simulink model "Quadcopter_V5"  (R2024a)
settings: Solver=ode4  StartTime=0.0  StopTime=inf  FixedStep=0.01  RelTol=1e-3
undefined symbols (not defined in the file): F, MIL, Severe
libraries: slpidlib x8, simulink_extras x4, aerolibpropulsion2 x4, aerolibwind2 x2, shared6dof x1, aerolibatmos2 x1, aerolibanimutils x1, sharedtransform x1, uavutilslib x1
(part 1 of 2)
settings Model: Creator=aceco  LastModifiedBy=Anthony

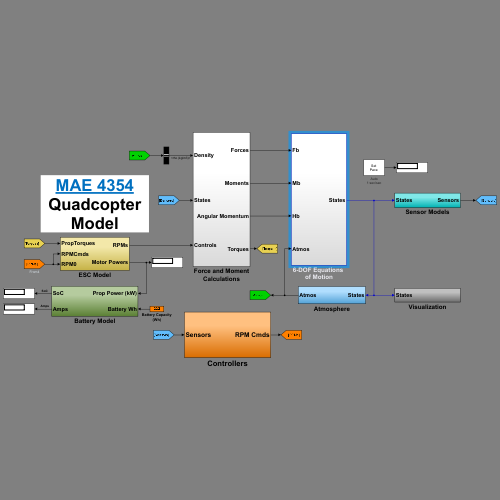
[thumbnail: Simulink's stored preview of the top-level diagram]
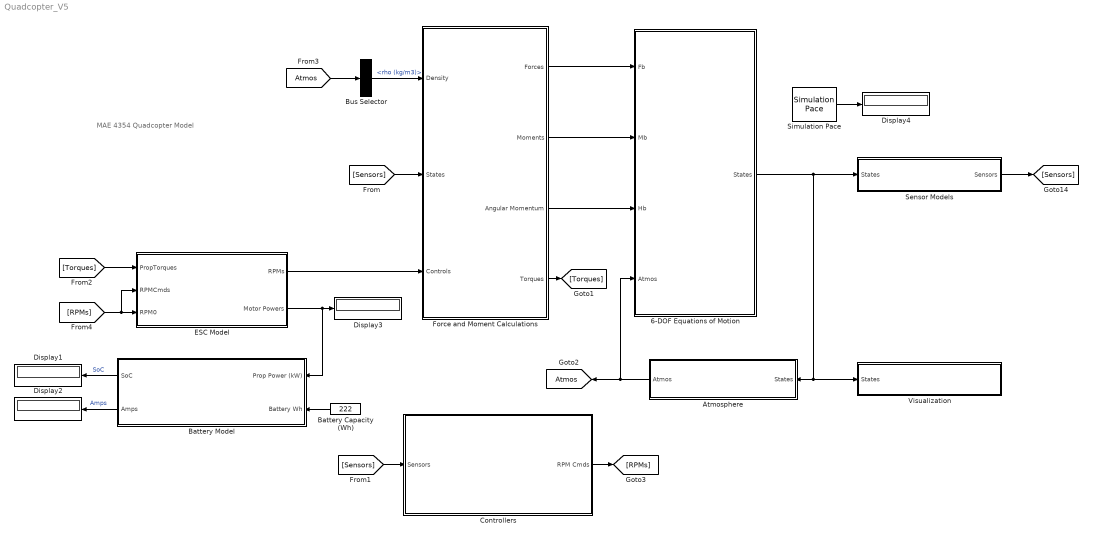
== system Quadcopter_V5 ==
  note: MAE 4354
      | Quadcopter Model
  6-DOF Equations of Motion : Subsystem
  Atmosphere : Subsystem
  Battery Capacity (Wh) : Constant  Value=222
  Battery Model : Subsystem
  Bus Selector : BusSelector  OutputSignals=rho (kg/m3)
  Controllers : Subsystem
  Display{1..4} (4 alike) : Display
  ESC Model : Subsystem
  Force and Moment Calculations : Subsystem
  Sensor Models : Subsystem
  Simulation Pace : aerolibanimutils/Simulation Pace  SimulationPace=1  SleepMode=Auto  OutputPaceError=on  SampleTime=-1
  Visualization : Subsystem
  tag scope: Atmos=global
  wires:
  Simulation Pace/1 -> Display4/1
  6-DOF Equations of Motion/1(States) -> Visualization/1(States), Atmosphere/1(States), Sensor Models/1(States)
  Force and Moment Calculations/1(Forces) -> 6-DOF Equations of Motion/1(Fb)
  Force and Moment Calculations/2(Moments) -> 6-DOF Equations of Motion/2(Mb)
  [Sensors] -> Force and Moment Calculations/2(States)
  ESC Model/1(RPMs) -> Force and Moment Calculations/3(Controls)
  [RPMs] -> ESC Model/2(RPMCmds), ESC Model/3(RPM0)
  Battery Model/2(Amps) -> Display2/1  "Amps"
  Battery Model/1(SoC) -> Display1/1  "SoC"
  Battery Capacity (Wh)/1 -> Battery Model/2(Battery Wh)
  ESC Model/2(Motor Powers) -> Display3/1, Battery Model/1(Prop Power (kW))
  Sensor Models/1(Sensors) -> [Sensors]
  [Sensors] -> Controllers/1(Sensors)
  Force and Moment Calculations/4(Torques) -> [Torques]
  [Torques] -> ESC Model/1(PropTorques)
  Atmosphere/1(Atmos) -> [Atmos], 6-DOF Equations of Motion/4(Atmos)
  Bus Selector/1 -> Force and Moment Calculations/1(Density)  "<rho (kg/m3)>"
  [Atmos] -> Bus Selector/1
  Force and Moment Calculations/3(Angular Momentum) -> 6-DOF Equations of Motion/3(Hb)
  Controllers/1(RPM Cmds) -> [RPMs]

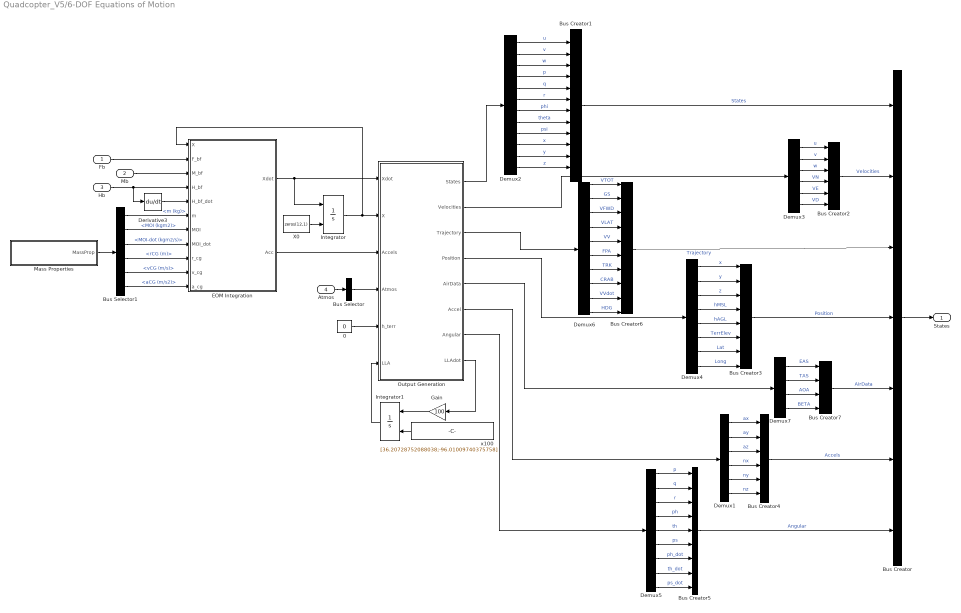
== system Quadcopter_V5/6-DOF Equations of Motion ==
  Fb : Inport
  Mb : Inport  Port=2
  Hb : Inport  Port=3
  Atmos : Inport  Port=4
  0 : Constant  Value=0
  Bus Creator : BusCreator  Inputs=7
  Bus Creator1 : BusCreator  Inputs=12
  Bus Creator2 : BusCreator  Inputs=6
  Bus Creator3 : BusCreator  Inputs=8
  Bus Creator4 : BusCreator  Inputs=6
  Bus Creator5 : BusCreator  Inputs=9
  Bus Creator6 : BusCreator  Inputs=10
  Bus Creator7 : BusCreator  Inputs=4
  Bus Selector : BusSelector  OutputSignals=V_wind (m/s),Om_wind (m/s),rho (kg/m3)  OutputAsBus=on
  Bus Selector1 : BusSelector  OutputSignals=m (kg),MOI (kgm2),MOI-dot (kgm2/s),rCG (m),vCG (m/s),aCG (m/s2)
  Demux1 : Demux  Outputs=6
  Demux2 : Demux  Outputs=12
  Demux3 : Demux  Outputs=6
  Demux4 : Demux  Outputs=8
  Demux5 : Demux  Outputs=9
  Demux6 : Demux  Outputs=10
  Demux7 : Demux
  Derivative3 : Derivative
  EOM Integration : MATLAB Function  TreatAsAtomicUnit=on
  Gain : Gain  Gain=100
  Integrator : Integrator  InitialConditionSource=external
  Integrator1 : Integrator  InitialConditionSource=external
  Mass Properties : Subsystem
  Output Generation : MATLAB Function  TreatAsAtomicUnit=on
  X0 : Constant  Value=zeros(12,1)
  x100 : Constant  Value=[36.20728752088038;-96.01009740375758]
  States : Outport  VectorParamsAs1DForOutWhenUnconnected=off
  wires:
  Bus Creator/1 -> States/1
  X0/1 -> Integrator/2
  Fb/1 -> EOM Integration/2(F_bf)
  Integrator/1 -> EOM Integration/1(X), Output Generation/2(X)
  Mb/1 -> EOM Integration/3(M_bf)
  Demux2/1 -> Bus Creator1/1  "u"
  Demux2/2 -> Bus Creator1/2  "v"
  Demux2/3 -> Bus Creator1/3  "w"
  Bus Creator1/1 -> Bus Creator/1  "States"
  Bus Creator2/1 -> Bus Creator/2  "Velocities"
  Demux3/3 -> Bus Creator2/3  "w"
  Demux3/2 -> Bus Creator2/2  "v"
  Demux3/1 -> Bus Creator2/1  "u"
  Demux2/4 -> Bus Creator1/4  "p"
  Demux2/5 -> Bus Creator1/5  "q"
  Demux2/6 -> Bus Creator1/6  "r"
  Demux3/4 -> Bus Creator2/4  "VN"
  Demux3/5 -> Bus Creator2/5  "VE"
  Demux3/6 -> Bus Creator2/6  "VD"
  Demux4/1 -> Bus Creator3/1  "x"
  Demux4/2 -> Bus Creator3/2  "y"
  Demux4/3 -> Bus Creator3/3  "z"
  Bus Creator3/1 -> Bus Creator/4  "Position"
  Demux1/1 -> Bus Creator4/1  "ax"
  Demux1/2 -> Bus Creator4/2  "ay"
  Demux1/3 -> Bus Creator4/3  "az"
  Demux1/4 -> Bus Creator4/4  "nx"
  Demux1/5 -> Bus Creator4/5  "ny"
  Demux1/6 -> Bus Creator4/6  "nz"
  Bus Creator4/1 -> Bus Creator/6  "Accels"
  Demux5/1 -> Bus Creator5/1  "p"
  Demux5/2 -> Bus Creator5/2  "q"
  Demux5/3 -> Bus Creator5/3  "r"
  Demux5/4 -> Bus Creator5/4  "ph"
  Demux5/5 -> Bus Creator5/5  "th"
  Demux5/6 -> Bus Creator5/6  "ps"
  Demux5/7 -> Bus Creator5/7  "ph_dot"
  Demux5/8 -> Bus Creator5/8  "th_dot"
  Demux5/9 -> Bus Creator5/9  "ps_dot"
  Bus Creator5/1 -> Bus Creator/7  "Angular"
  Bus Creator7/1 -> Bus Creator/5  "AirData"
  Bus Creator6/1 -> Bus Creator/3  "Trajectory"
  EOM Integration/1(Xdot) -> Integrator/1, Output Generation/1(Xdot)
  Demux4/8 -> Bus Creator3/8  "Long"
  Demux4/7 -> Bus Creator3/7  "Lat"
  Demux4/6 -> Bus Creator3/6  "TerrElev"
  Demux4/5 -> Bus Creator3/5  "hAGL"
  Demux4/4 -> Bus Creator3/4  "hMSL"
  EOM Integration/2(Acc) -> Output Generation/3(Accels)
  Atmos/1 -> Bus Selector/1
  Bus Selector/1 -> Output Generation/4(Atmos)
  Output Generation/8(LLAdot) -> Gain/1
  Integrator1/1 -> Output Generation/6(LLA)
  x100/1 -> Integrator1/2
  Output Generation/1(States) -> Demux2/1
  Demux2/7 -> Bus Creator1/7  "phi"
  Demux2/8 -> Bus Creator1/8  "theta"
  Demux2/9 -> Bus Creator1/9  "psi"
  Demux2/10 -> Bus Creator1/10  "x"
  Demux2/11 -> Bus Creator1/11  "y"
  Demux2/12 -> Bus Creator1/12  "z"
  Output Generation/2(Velocities) -> Demux3/1
  Demux6/7 -> Bus Creator6/7  "TRK"
  Demux6/8 -> Bus Creator6/8  "CRAB"
  Demux6/9 -> Bus Creator6/9  "VVdot"
  Demux6/1 -> Bus Creator6/1  "VTOT"
  Demux6/4 -> Bus Creator6/4  "VLAT"
  Demux6/5 -> Bus Creator6/5  "VV"
  Demux6/3 -> Bus Creator6/3  "VFWD"
  Demux6/2 -> Bus Creator6/2  "GS"
  Demux6/6 -> Bus Creator6/6  "FPA"
  Demux6/10 -> Bus Creator6/10  "HDG"
  Output Generation/3(Trajectory) -> Demux6/1
  Output Generation/4(Position) -> Demux4/1
  Demux7/4 -> Bus Creator7/4  "BETA"
  Demux7/1 -> Bus Creator7/1  "EAS"
  Demux7/2 -> Bus Creator7/2  "TAS"
  Demux7/3 -> Bus Creator7/3  "AOA"
  Output Generation/5(AirData) -> Demux7/1
  Output Generation/6(Accel) -> Demux1/1
  Output Generation/7(Angular) -> Demux5/1
  0/1 -> Output Generation/5(h_terr)
  Gain/1 -> Integrator1/1
  Hb/1 -> EOM Integration/4(H_bf), Derivative3/1
  Derivative3/1 -> EOM Integration/5(H_bf_dot)
  Mass Properties/1(MassProp) -> Bus Selector1/1
  Bus Selector1/1 -> EOM Integration/6(m)  "<m (kg)>"
  Bus Selector1/4 -> EOM Integration/9(r_cg)  "<rCG (m)>"
  Bus Selector1/5 -> EOM Integration/10(v_cg)  "<vCG (m/s)>"
  Bus Selector1/6 -> EOM Integration/11(a_cg)  "<aCG (m/s2)>"
  Bus Selector1/2 -> EOM Integration/7(MOI)  "<MOI (kgm2)>"
  Bus Selector1/3 -> EOM Integration/8(MOI_dot)  "<MOI-dot (kgm2/s)>"

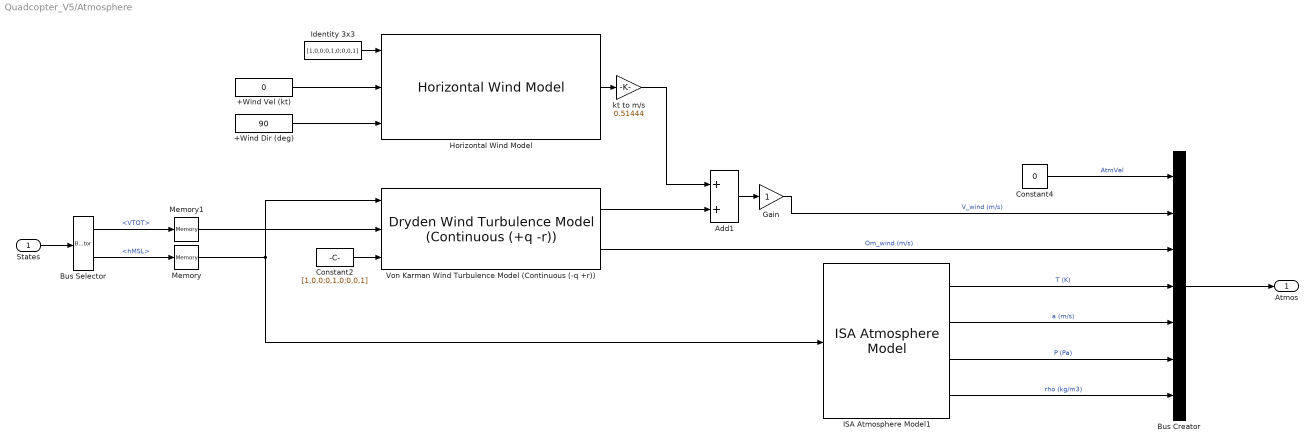
== system Quadcopter_V5/Atmosphere ==
  States : Inport
  +Wind Dir (deg) : Constant  Value=90
  +Wind Vel (kt) : Constant  Value=0
  Add1 : Sum  Inputs=2
  Bus Creator : BusCreator  Inputs=7
  Bus Selector : BusSelector  OutputSignals=Trajectory.VTOT,Position.hMSL
  Constant2 : Constant  Value=[1,0,0;0,1,0;0,0,1]
  Constant4 : Constant  Value=0
  Gain : Gain
  Horizontal Wind Model : aerolibwind2/Horizontal Wind Model  units=English (Velocity in kts)  Vw_source=External  Vwind=Init.WindSpd  W_source=External  Wdeg=Init.WindDir
  ISA Atmosphere Model1 : aerolibatmos2/ISA Atmosphere Model  useExtended=off  action=Warning  custom=off  viscosityOut=off  g=9.80665  gamma=1.4  R=287.0531  L=0.0065  h_trop=11000  h_strat=20000  rho0=1.225  P0=101325  T0=288.15  h0=0  S=110.4  Tref=273.15  muref=1.716e-5
  Identity 3x3 : Constant  Value=[1,0,0;0,1,0;0,0,1]
  Memory : Memory
  Memory1 : Memory
  Von Karman Wind Turbulence Model (Continuous (-q +r)) : aerolibwind2/Dryden Wind Turbulence Model  (Continuous (+q -r))  units=Metric (MKS)  spec=MIL-F-8785C  model=Continuous Von Karman (-q +r)  W20=3  Wdeg=90  TurbProb=10^-5 - Severe  L_high=762  Wingspan=2  ts=0.2  Seed=[23341 23342 23343 23344]  T_on=off
  kt to m/s : Gain  Gain=0.51444
  Atmos : Outport  VectorParamsAs1DForOutWhenUnconnected=off
  wires:
  States/1 -> Bus Selector/1
  Bus Selector/2 -> Memory/1  "<hMSL>"
  Horizontal Wind Model/1 -> kt to m/s/1
  Add1/1 -> Gain/1
  ISA Atmosphere Model1/1 -> Bus Creator/4  "T (K)"
  ISA Atmosphere Model1/2 -> Bus Creator/5  "a (m/s)"
  ISA Atmosphere Model1/3 -> Bus Creator/6  "P (Pa)"
  ISA Atmosphere Model1/4 -> Bus Creator/7  "rho (kg/m3)"
  Bus Creator/1 -> Atmos/1
  Von Karman Wind Turbulence Model (Continuous (-q +r))/1 -> Add1/2
  Von Karman Wind Turbulence Model (Continuous (-q +r))/2 -> Bus Creator/3  "Om_wind (m/s)"
  Constant4/1 -> Bus Creator/1  "AtmVel"
  Identity 3x3/1 -> Horizontal Wind Model/1
  Constant2/1 -> Von Karman Wind Turbulence Model (Continuous (-q +r))/3
  kt to m/s/1 -> Add1/1
  +Wind Vel (kt)/1 -> Horizontal Wind Model/2
  +Wind Dir (deg)/1 -> Horizontal Wind Model/3
  Bus Selector/1 -> Memory1/1  "<VTOT>"
  Gain/1 -> Bus Creator/2  "V_wind (m/s)"
  Memory/1 -> Von Karman Wind Turbulence Model (Continuous (-q +r))/1, ISA Atmosphere Model1/1
  Memory1/1 -> Von Karman Wind Turbulence Model (Continuous (-q +r))/2

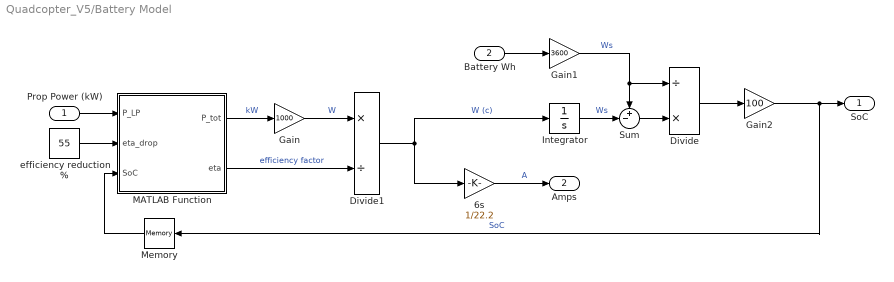
== system Quadcopter_V5/Battery Model ==
  Prop Power (kW) : Inport
  Battery Wh : Inport  Port=2
  6s : Gain  Gain=1/22.2
  Divide : Product  Inputs=/*
  Divide1 : Product  Inputs=*/
  Gain : Gain  Gain=1000
  Gain1 : Gain  Gain=3600
  Gain2 : Gain  Gain=100
  Integrator : Integrator
  MATLAB Function : MATLAB Function  TreatAsAtomicUnit=on
  Memory : Memory  InitialCondition=100
  Sum : Sum  Inputs=+-|
  efficiency reduction % : Constant  Value=55
  SoC : Outport
  Amps : Outport  Port=2
  wires:
  Battery Wh/1 -> Gain1/1
  6s/1 -> Amps/1  "A"
  Prop Power (kW)/1 -> MATLAB Function/1(P_LP)
  MATLAB Function/1(P_tot) -> Gain/1  "kW"
  Sum/1 -> Divide/2
  Integrator/1 -> Sum/2  "Ws"
  Divide/1 -> Gain2/1
  Gain2/1 -> Memory/1, SoC/1  "SoC"
  Divide1/1 -> 6s/1, Integrator/1  "W (c)"
  Gain1/1 -> Sum/1, Divide/1  "Ws"
  Gain/1 -> Divide1/1  "W"
  MATLAB Function/2(eta) -> Divide1/2  "efficiency factor"
  Memory/1 -> MATLAB Function/3(SoC)
  efficiency reduction %/1 -> MATLAB Function/2(eta_drop)

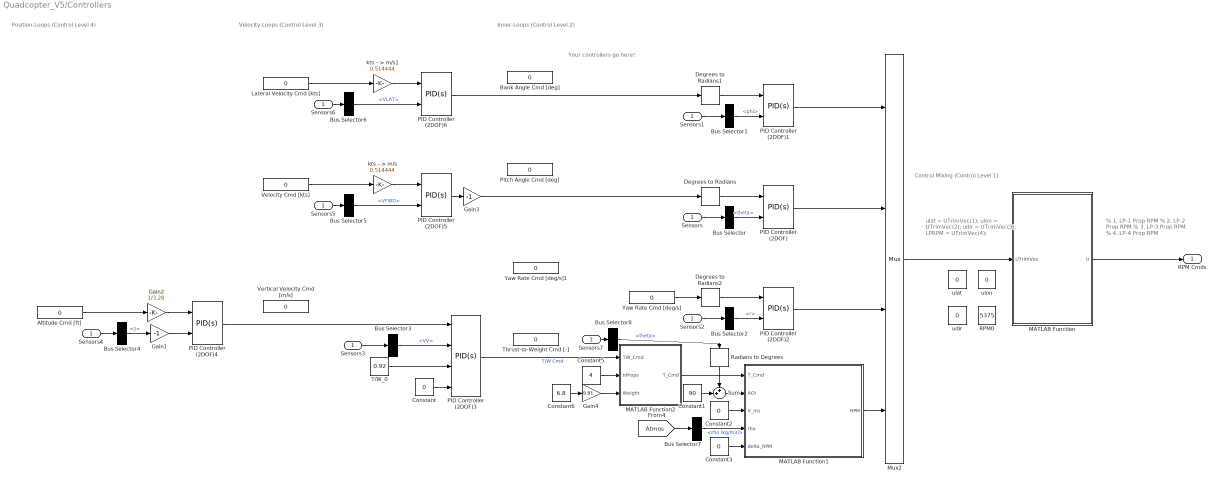
== system Quadcopter_V5/Controllers ==
  note: Inner-Loops (Control Level 2)
  note: Control Mixing (Control Level 1)
  note: Your controllers go here!
  note: ulat = UTrimVec(1);
      | ulon = UTrimVec(2);
      | udir = UTrimVec(3);
      | LPRPM = UTrimVec(4);
  note: % 1. LP-1 Prop RPM
      | % 2. LP-2 Prop RPM
      | % 3. LP-3 Prop RPM
      | % 4. LP-4 Prop RPM
  note: Velocity-Loops (Control Level 3)
  note: Position-Loops (Control Level 4)
  Sensors : Inport
  Altitude Cmd [ft] : Constant  Value=0
  Bank Angle Cmd [deg] : Constant  Value=0
  Bus Selector : BusSelector  OutputSignals=theta
  Bus Selector1 : BusSelector  OutputSignals=phi
  Bus Selector2 : BusSelector  OutputSignals=r
  Bus Selector3 : BusSelector  OutputSignals=VV
  Bus Selector4 : BusSelector  OutputSignals=z
  Bus Selector5 : BusSelector  OutputSignals=VFWD
  Bus Selector6 : BusSelector  OutputSignals=VLAT
  Bus Selector7 : BusSelector  OutputSignals=rho (kg/m3)
  Bus Selector8 : BusSelector  OutputSignals=theta
  Constant : Constant  Value=0
  Constant1 : Constant  Value=90
  Constant2 : Constant  Value=0
  Constant3 : Constant  Value=0
  Constant5 : Constant  Value=4
  Constant6 : Constant  Value=6.8
  Degrees to Radians : simulink_extras/Transformations/Degrees to Radians
  Degrees to Radians1 : simulink_extras/Transformations/Degrees to Radians
  Degrees to Radians2 : simulink_extras/Transformations/Degrees to Radians
  Gain1 : Gain  Gain=-1
  Gain2 : Gain  Gain=1/3.28
  Gain3 : Gain  Gain=-1
  Gain4 : Gain  Gain=9.81
  Lateral Velocity Cmd [kts] : Constant  Value=0
  MATLAB Function : MATLAB Function  TreatAsAtomicUnit=on
  MATLAB Function1 : MATLAB Function  TreatAsAtomicUnit=on
  MATLAB Function2 : MATLAB Function  TreatAsAtomicUnit=on
  Mux2 : Mux
  PID Controller (2DOF) : slpidlib/PID Controller (2DOF)  Controller=PID  Form=Parallel  TimeDomain=Continuous-time  UseExternalTs=off  SampleTime=-1  IntegratorMethod=Forward Euler  FilterMethod=Forward Euler  ControllerParametersSource=internal  P=2  I=0.5  UseKiTs=off  D=1  UseExternalDerivativeSource=off  N=100  UseFilter=on  b=1  c=1  TunerSelectOption=Transfer Function Based (PID Tuner App)  InitialConditionSource=internal  InitialConditionForIntegrator=0  InitialConditionForFilter=0  DifferentiatorICPrevScaledInput=0  ExternalReset=none  TrackingMode=off  Kt=1  LimitOutput=on  SatLimitsSource=internal  UpperSaturationLimit=1  LowerSaturationLimit=-1  LinearizeAsGain=on  AntiWindupMode=clamping  Kb=1  LimitIntegrator=off  UpperIntegratorSaturationLimit=inf  LowerIntegratorSaturationLimit=-inf  POutMin=[]  POutMax=[]  IOutMin=[]  IOutMax=[]  DOutMin=[]  DOutMax=[]  NOutMin=[]  NOutMax=[]  bOutMin=[]  bOutMax=[]  cOutMin=[]  cOutMax=[]  SumOutMin=[]  SumOutMax=[]  SaturationOutMin=[]  SaturationOutMax=[]  PParamMin=[]  PParamMax=[]  IParamMin=[]  IParamMax=[]  DParamMin=[]  DParamMax=[]  NParamMin=[]  NParamMax=[]  bParamMin=[]  bParamMax=[]  cParamMin=[]  cParamMax=[]  KbParamMin=[]  KbParamMax=[]  KtParamMin=[]  KtParamMax=[]  KbOutMin=[]  KbOutMax=[]  KtOutMin=[]  KtOutMax=[]  IntegratorOutMin=[]  IntegratorOutMax=[]  FilterOutMin=[]  FilterOutMax=[]  SumI1OutMin=[]  SumI1OutMax=[]  SumI2OutMin=[]  SumI2OutMax=[]  SumI3OutMin=[]  SumI3OutMax=[]  SumI4OutMin=[]  SumI4OutMax=[]  SumDOutMin=[]  SumDOutMax=[]  Sum1OutMin=[]  Sum1OutMax=[]  Sum2OutMin=[]  Sum2OutMax=[]  Sum3OutMin=[]  Sum3OutMax=[]  DifferentiatorOutMin=[]  DifferentiatorOutMax=[]  FilterDiffOutCoefMin=[]  FilterDiffOutCoefMax=[]  ReciprocalOutMin=[]  ReciprocalOutMax=[]  SumDenOutMin=[]  SumDenOutMax=[]  SumNumOutMin=[]  SumNumOutMax=[]  DivideOutMin=[]  DivideOutMax=[]  UdiffTsProdOutMin=[]  UdiffTsProdOutMax=[]  NTsProdOutMin=[]  NTsProdOutMax=[]  UintegralTsProdOutMin=[]  UintegralTsProdOutMax=[]  UngainTsProdOutMin=[]  UngainTsProdOutMax=[]  ClampingZeroOutDataTypeStr=Inherit: Inherit via back propagation  ClampingZeroOutMin=[]  ClampingZeroOutMax=[]  FilterDenConstantOutDataTypeStr=Inherit: Inherit via back propagation  FilterDenConstantOutMin=[]  FilterDenConstantOutMax=[]  PCopyOutDataTypeStr=Inherit: Inherit via back propagation  PCopyOutMin=[]  PCopyOutMax=[]  NCopyOutDataTypeStr=Inherit: Inherit via back propagation  NCopyOutMin=[]  NCopyOutMax=[]  IntegratorContinuousStateAttributes=''  IntegratorStateMustResolveToSignalObject=off  IntegratorRTWStateStorageClass=Auto  FilterContinuousStateAttributes=''  FilterStateMustResolveToSignalObject=off  FilterRTWStateStorageClass=Auto  ParallelPVariant=InternalParameters  IdealPVariant=Disabled  IVariant=InternalParameters  DVariant=InternalParameters  bVariant=InternalParameters  cVariant=InternalParameters  IntegratorVariant=Continuous  SatVariant=Enabled  AWVariant=ContClampingParallel  PCopyVariant=Disabled  TRVariant=Disabled  FdbkBlocksVariant=Forward  IdealPFdbkVariant=Disabled  SatFdbkVariant=Disabled  DerivativeFilterVariant=ContFilter  NVariant=InternalParameters  NCopyVariant=Disabled  FilterICVariant=InternalICsFilter  IntegratorICVariant=InternalICs  ExternalResetVariant=Disabled  TRSumVariant=Passthrough  SumFdbkVariant=Disabled  SumVariant=Sum_PID  TsampFilterVariant=InternalTs  TsampNgainVariant=Passthrough  TsampIntegralVariant=Disabled_SignalSpec  ExternalSaturationOutDataTypeStr=Inherit: Same as second input  DerivativeSourceVariant=ErrorSignal
  PID Controller (2DOF)1 : slpidlib/PID Controller (2DOF)  Controller=PID  Form=Parallel  TimeDomain=Continuous-time  UseExternalTs=off  SampleTime=-1  IntegratorMethod=Forward Euler  FilterMethod=Forward Euler  ControllerParametersSource=internal  P=2  I=0.5  UseKiTs=off  D=1  UseExternalDerivativeSource=off  N=100  UseFilter=on  b=1  c=1  TunerSelectOption=Transfer Function Based (PID Tuner App)  InitialConditionSource=internal  InitialConditionForIntegrator=0  InitialConditionForFilter=0  DifferentiatorICPrevScaledInput=0  ExternalReset=none  TrackingMode=off  Kt=1  LimitOutput=on  SatLimitsSource=internal  UpperSaturationLimit=1  LowerSaturationLimit=-1  LinearizeAsGain=on  AntiWindupMode=clamping  Kb=1  LimitIntegrator=off  UpperIntegratorSaturationLimit=inf  LowerIntegratorSaturationLimit=-inf  POutMin=[]  POutMax=[]  IOutMin=[]  IOutMax=[]  DOutMin=[]  DOutMax=[]  NOutMin=[]  NOutMax=[]  bOutMin=[]  bOutMax=[]  cOutMin=[]  cOutMax=[]  SumOutMin=[]  SumOutMax=[]  SaturationOutMin=[]  SaturationOutMax=[]  PParamMin=[]  PParamMax=[]  IParamMin=[]  IParamMax=[]  DParamMin=[]  DParamMax=[]  NParamMin=[]  NParamMax=[]  bParamMin=[]  bParamMax=[]  cParamMin=[]  cParamMax=[]  KbParamMin=[]  KbParamMax=[]  KtParamMin=[]  KtParamMax=[]  KbOutMin=[]  KbOutMax=[]  KtOutMin=[]  KtOutMax=[]  IntegratorOutMin=[]  IntegratorOutMax=[]  FilterOutMin=[]  FilterOutMax=[]  SumI1OutMin=[]  SumI1OutMax=[]  SumI2OutMin=[]  SumI2OutMax=[]  SumI3OutMin=[]  SumI3OutMax=[]  SumI4OutMin=[]  SumI4OutMax=[]  SumDOutMin=[]  SumDOutMax=[]  Sum1OutMin=[]  Sum1OutMax=[]  Sum2OutMin=[]  Sum2OutMax=[]  Sum3OutMin=[]  Sum3OutMax=[]  DifferentiatorOutMin=[]  DifferentiatorOutMax=[]  FilterDiffOutCoefMin=[]  FilterDiffOutCoefMax=[]  ReciprocalOutMin=[]  ReciprocalOutMax=[]  SumDenOutMin=[]  SumDenOutMax=[]  SumNumOutMin=[]  SumNumOutMax=[]  DivideOutMin=[]  DivideOutMax=[]  UdiffTsProdOutMin=[]  UdiffTsProdOutMax=[]  NTsProdOutMin=[]  NTsProdOutMax=[]  UintegralTsProdOutMin=[]  UintegralTsProdOutMax=[]  UngainTsProdOutMin=[]  UngainTsProdOutMax=[]  ClampingZeroOutDataTypeStr=Inherit: Inherit via back propagation  ClampingZeroOutMin=[]  ClampingZeroOutMax=[]  FilterDenConstantOutDataTypeStr=Inherit: Inherit via back propagation  FilterDenConstantOutMin=[]  FilterDenConstantOutMax=[]  PCopyOutDataTypeStr=Inherit: Inherit via back propagation  PCopyOutMin=[]  PCopyOutMax=[]  NCopyOutDataTypeStr=Inherit: Inherit via back propagation  NCopyOutMin=[]  NCopyOutMax=[]  IntegratorContinuousStateAttributes=''  IntegratorStateMustResolveToSignalObject=off  IntegratorRTWStateStorageClass=Auto  FilterContinuousStateAttributes=''  FilterStateMustResolveToSignalObject=off  FilterRTWStateStorageClass=Auto  ParallelPVariant=InternalParameters  IdealPVariant=Disabled  IVariant=InternalParameters  DVariant=InternalParameters  bVariant=InternalParameters  cVariant=InternalParameters  IntegratorVariant=Continuous  SatVariant=Enabled  AWVariant=ContClampingParallel  PCopyVariant=Disabled  TRVariant=Disabled  FdbkBlocksVariant=Forward  IdealPFdbkVariant=Disabled  SatFdbkVariant=Disabled  DerivativeFilterVariant=ContFilter  NVariant=InternalParameters  NCopyVariant=Disabled  FilterICVariant=InternalICsFilter  IntegratorICVariant=InternalICs  ExternalResetVariant=Disabled  TRSumVariant=Passthrough  SumFdbkVariant=Disabled  SumVariant=Sum_PID  TsampFilterVariant=InternalTs  TsampNgainVariant=Passthrough  TsampIntegralVariant=Disabled_SignalSpec  ExternalSaturationOutDataTypeStr=Inherit: Same as second input  DerivativeSourceVariant=ErrorSignal
  PID Controller (2DOF)2 : slpidlib/PID Controller (2DOF)  Controller=PID  Form=Parallel  TimeDomain=Continuous-time  UseExternalTs=off  SampleTime=-1  IntegratorMethod=Forward Euler  FilterMethod=Forward Euler  ControllerParametersSource=internal  P=2  I=0.5  UseKiTs=off  D=0  UseExternalDerivativeSource=off  N=100  UseFilter=on  b=1  c=1  TunerSelectOption=Transfer Function Based (PID Tuner App)  InitialConditionSource=internal  InitialConditionForIntegrator=0  InitialConditionForFilter=0  DifferentiatorICPrevScaledInput=0  ExternalReset=none  TrackingMode=off  Kt=1  LimitOutput=on  SatLimitsSource=internal  UpperSaturationLimit=1  LowerSaturationLimit=-1  LinearizeAsGain=on  AntiWindupMode=clamping  Kb=1  LimitIntegrator=off  UpperIntegratorSaturationLimit=inf  LowerIntegratorSaturationLimit=-inf  POutMin=[]  POutMax=[]  IOutMin=[]  IOutMax=[]  DOutMin=[]  DOutMax=[]  NOutMin=[]  NOutMax=[]  bOutMin=[]  bOutMax=[]  cOutMin=[]  cOutMax=[]  SumOutMin=[]  SumOutMax=[]  SaturationOutMin=[]  SaturationOutMax=[]  PParamMin=[]  PParamMax=[]  IParamMin=[]  IParamMax=[]  DParamMin=[]  DParamMax=[]  NParamMin=[]  NParamMax=[]  bParamMin=[]  bParamMax=[]  cParamMin=[]  cParamMax=[]  KbParamMin=[]  KbParamMax=[]  KtParamMin=[]  KtParamMax=[]  KbOutMin=[]  KbOutMax=[]  KtOutMin=[]  KtOutMax=[]  IntegratorOutMin=[]  IntegratorOutMax=[]  FilterOutMin=[]  FilterOutMax=[]  SumI1OutMin=[]  SumI1OutMax=[]  SumI2OutMin=[]  SumI2OutMax=[]  SumI3OutMin=[]  SumI3OutMax=[]  SumI4OutMin=[]  SumI4OutMax=[]  SumDOutMin=[]  SumDOutMax=[]  Sum1OutMin=[]  Sum1OutMax=[]  Sum2OutMin=[]  Sum2OutMax=[]  Sum3OutMin=[]  Sum3OutMax=[]  DifferentiatorOutMin=[]  DifferentiatorOutMax=[]  FilterDiffOutCoefMin=[]  FilterDiffOutCoefMax=[]  ReciprocalOutMin=[]  ReciprocalOutMax=[]  SumDenOutMin=[]  SumDenOutMax=[]  SumNumOutMin=[]  SumNumOutMax=[]  DivideOutMin=[]  DivideOutMax=[]  UdiffTsProdOutMin=[]  UdiffTsProdOutMax=[]  NTsProdOutMin=[]  NTsProdOutMax=[]  UintegralTsProdOutMin=[]  UintegralTsProdOutMax=[]  UngainTsProdOutMin=[]  UngainTsProdOutMax=[]  ClampingZeroOutDataTypeStr=Inherit: Inherit via back propagation  ClampingZeroOutMin=[]  ClampingZeroOutMax=[]  FilterDenConstantOutDataTypeStr=Inherit: Inherit via back propagation  FilterDenConstantOutMin=[]  FilterDenConstantOutMax=[]  PCopyOutDataTypeStr=Inherit: Inherit via back propagation  PCopyOutMin=[]  PCopyOutMax=[]  NCopyOutDataTypeStr=Inherit: Inherit via back propagation  NCopyOutMin=[]  NCopyOutMax=[]  IntegratorContinuousStateAttributes=''  IntegratorStateMustResolveToSignalObject=off  IntegratorRTWStateStorageClass=Auto  FilterContinuousStateAttributes=''  FilterStateMustResolveToSignalObject=off  FilterRTWStateStorageClass=Auto  ParallelPVariant=InternalParameters  IdealPVariant=Disabled  IVariant=InternalParameters  DVariant=InternalParameters  bVariant=InternalParameters  cVariant=InternalParameters  IntegratorVariant=Continuous  SatVariant=Enabled  AWVariant=ContClampingParallel  PCopyVariant=Disabled  TRVariant=Disabled  FdbkBlocksVariant=Forward  IdealPFdbkVariant=Disabled  SatFdbkVariant=Disabled  DerivativeFilterVariant=ContFilter  NVariant=InternalParameters  NCopyVariant=Disabled  FilterICVariant=InternalICsFilter  IntegratorICVariant=InternalICs  ExternalResetVariant=Disabled  TRSumVariant=Passthrough  SumFdbkVariant=Disabled  SumVariant=Sum_PID  TsampFilterVariant=InternalTs  TsampNgainVariant=Passthrough  TsampIntegralVariant=Disabled_SignalSpec  ExternalSaturationOutDataTypeStr=Inherit: Same as second input  DerivativeSourceVariant=ErrorSignal
  PID Controller (2DOF)3 : slpidlib/PID Controller (2DOF)  Controller=PID  Form=Parallel  TimeDomain=Continuous-time  UseExternalTs=off  SampleTime=-1  IntegratorMethod=Forward Euler  FilterMethod=Forward Euler  ControllerParametersSource=internal  P=0.5  I=0.25  UseKiTs=off  D=0  UseExternalDerivativeSource=off  N=100  UseFilter=on  b=1  c=1  TunerSelectOption=Transfer Function Based (PID Tuner App)  InitialConditionSource=external  InitialConditionForIntegrator=0  InitialConditionForFilter=0  DifferentiatorICPrevScaledInput=0  ExternalReset=none  TrackingMode=off  Kt=1  LimitOutput=on  SatLimitsSource=internal  UpperSaturationLimit=1.5  LowerSaturationLimit=0  LinearizeAsGain=on  AntiWindupMode=clamping  Kb=1  LimitIntegrator=off  UpperIntegratorSaturationLimit=inf  LowerIntegratorSaturationLimit=-inf  POutMin=[]  POutMax=[]  IOutMin=[]  IOutMax=[]  DOutMin=[]  DOutMax=[]  NOutMin=[]  NOutMax=[]  bOutMin=[]  bOutMax=[]  cOutMin=[]  cOutMax=[]  SumOutMin=[]  SumOutMax=[]  SaturationOutMin=[]  SaturationOutMax=[]  PParamMin=[]  PParamMax=[]  IParamMin=[]  IParamMax=[]  DParamMin=[]  DParamMax=[]  NParamMin=[]  NParamMax=[]  bParamMin=[]  bParamMax=[]  cParamMin=[]  cParamMax=[]  KbParamMin=[]  KbParamMax=[]  KtParamMin=[]  KtParamMax=[]  KbOutMin=[]  KbOutMax=[]  KtOutMin=[]  KtOutMax=[]  IntegratorOutMin=[]  IntegratorOutMax=[]  FilterOutMin=[]  FilterOutMax=[]  SumI1OutMin=[]  SumI1OutMax=[]  SumI2OutMin=[]  SumI2OutMax=[]  SumI3OutMin=[]  SumI3OutMax=[]  SumI4OutMin=[]  SumI4OutMax=[]  SumDOutMin=[]  SumDOutMax=[]  Sum1OutMin=[]  Sum1OutMax=[]  Sum2OutMin=[]  Sum2OutMax=[]  Sum3OutMin=[]  Sum3OutMax=[]  DifferentiatorOutMin=[]  DifferentiatorOutMax=[]  FilterDiffOutCoefMin=[]  FilterDiffOutCoefMax=[]  ReciprocalOutMin=[]  ReciprocalOutMax=[]  SumDenOutMin=[]  SumDenOutMax=[]  SumNumOutMin=[]  SumNumOutMax=[]  DivideOutMin=[]  DivideOutMax=[]  UdiffTsProdOutMin=[]  UdiffTsProdOutMax=[]  NTsProdOutMin=[]  NTsProdOutMax=[]  UintegralTsProdOutMin=[]  UintegralTsProdOutMax=[]  UngainTsProdOutMin=[]  UngainTsProdOutMax=[]  ClampingZeroOutDataTypeStr=Inherit: Inherit via back propagation  ClampingZeroOutMin=[]  ClampingZeroOutMax=[]  FilterDenConstantOutDataTypeStr=Inherit: Inherit via back propagation  FilterDenConstantOutMin=[]  FilterDenConstantOutMax=[]  PCopyOutDataTypeStr=Inherit: Inherit via back propagation  PCopyOutMin=[]  PCopyOutMax=[]  NCopyOutDataTypeStr=Inherit: Inherit via back propagation  NCopyOutMin=[]  NCopyOutMax=[]  IntegratorContinuousStateAttributes=''  IntegratorStateMustResolveToSignalObject=off  IntegratorRTWStateStorageClass=Auto  FilterContinuousStateAttributes=''  FilterStateMustResolveToSignalObject=off  FilterRTWStateStorageClass=Auto  ParallelPVariant=InternalParameters  IdealPVariant=Disabled  IVariant=InternalParameters  DVariant=InternalParameters  bVariant=InternalParameters  cVariant=InternalParameters  IntegratorVariant=Continuous  SatVariant=Enabled  AWVariant=ContClampingParallel  PCopyVariant=Disabled  TRVariant=Disabled  FdbkBlocksVariant=Forward  IdealPFdbkVariant=Disabled  SatFdbkVariant=Disabled  DerivativeFilterVariant=ContFilter  NVariant=InternalParameters  NCopyVariant=Disabled  FilterICVariant=ExternalICs  IntegratorICVariant=ExternalICs  ExternalResetVariant=Disabled  TRSumVariant=Passthrough  SumFdbkVariant=Disabled  SumVariant=Sum_PID  TsampFilterVariant=InternalTs  TsampNgainVariant=Passthrough  TsampIntegralVariant=Disabled_SignalSpec  ExternalSaturationOutDataTypeStr=Inherit: Same as second input  DerivativeSourceVariant=ErrorSignal
  PID Controller (2DOF)4 : slpidlib/PID Controller (2DOF)  Controller=PID  Form=Parallel  TimeDomain=Continuous-time  UseExternalTs=off  SampleTime=-1  IntegratorMethod=Forward Euler  FilterMethod=Forward Euler  ControllerParametersSource=internal  P=0.5  I=0  UseKiTs=off  D=0  UseExternalDerivativeSource=off  N=100  UseFilter=on  b=1  c=1  TunerSelectOption=Transfer Function Based (PID Tuner App)  InitialConditionSource=internal  InitialConditionForIntegrator=0  InitialConditionForFilter=0  DifferentiatorICPrevScaledInput=0  ExternalReset=none  TrackingMode=off  Kt=1  LimitOutput=on  SatLimitsSource=internal  UpperSaturationLimit=5  LowerSaturationLimit=-5  LinearizeAsGain=on  AntiWindupMode=clamping  Kb=1  LimitIntegrator=off  UpperIntegratorSaturationLimit=inf  LowerIntegratorSaturationLimit=-inf  POutMin=[]  POutMax=[]  IOutMin=[]  IOutMax=[]  DOutMin=[]  DOutMax=[]  NOutMin=[]  NOutMax=[]  bOutMin=[]  bOutMax=[]  cOutMin=[]  cOutMax=[]  SumOutMin=[]  SumOutMax=[]  SaturationOutMin=[]  SaturationOutMax=[]  PParamMin=[]  PParamMax=[]  IParamMin=[]  IParamMax=[]  DParamMin=[]  DParamMax=[]  NParamMin=[]  NParamMax=[]  bParamMin=[]  bParamMax=[]  cParamMin=[]  cParamMax=[]  KbParamMin=[]  KbParamMax=[]  KtParamMin=[]  KtParamMax=[]  KbOutMin=[]  KbOutMax=[]  KtOutMin=[]  KtOutMax=[]  IntegratorOutMin=[]  IntegratorOutMax=[]  FilterOutMin=[]  FilterOutMax=[]  SumI1OutMin=[]  SumI1OutMax=[]  SumI2OutMin=[]  SumI2OutMax=[]  SumI3OutMin=[]  SumI3OutMax=[]  SumI4OutMin=[]  SumI4OutMax=[]  SumDOutMin=[]  SumDOutMax=[]  Sum1OutMin=[]  Sum1OutMax=[]  Sum2OutMin=[]  Sum2OutMax=[]  Sum3OutMin=[]  Sum3OutMax=[]  DifferentiatorOutMin=[]  DifferentiatorOutMax=[]  FilterDiffOutCoefMin=[]  FilterDiffOutCoefMax=[]  ReciprocalOutMin=[]  ReciprocalOutMax=[]  SumDenOutMin=[]  SumDenOutMax=[]  SumNumOutMin=[]  SumNumOutMax=[]  DivideOutMin=[]  DivideOutMax=[]  UdiffTsProdOutMin=[]  UdiffTsProdOutMax=[]  NTsProdOutMin=[]  NTsProdOutMax=[]  UintegralTsProdOutMin=[]  UintegralTsProdOutMax=[]  UngainTsProdOutMin=[]  UngainTsProdOutMax=[]  ClampingZeroOutDataTypeStr=Inherit: Inherit via back propagation  ClampingZeroOutMin=[]  ClampingZeroOutMax=[]  FilterDenConstantOutDataTypeStr=Inherit: Inherit via back propagation  FilterDenConstantOutMin=[]  FilterDenConstantOutMax=[]  PCopyOutDataTypeStr=Inherit: Inherit via back propagation  PCopyOutMin=[]  PCopyOutMax=[]  NCopyOutDataTypeStr=Inherit: Inherit via back propagation  NCopyOutMin=[]  NCopyOutMax=[]  IntegratorContinuousStateAttributes=''  IntegratorStateMustResolveToSignalObject=off  IntegratorRTWStateStorageClass=Auto  FilterContinuousStateAttributes=''  FilterStateMustResolveToSignalObject=off  FilterRTWStateStorageClass=Auto  ParallelPVariant=InternalParameters  IdealPVariant=Disabled  IVariant=InternalParameters  DVariant=InternalParameters  bVariant=InternalParameters  cVariant=InternalParameters  IntegratorVariant=Continuous  SatVariant=Enabled  AWVariant=ContClampingParallel  PCopyVariant=Disabled  TRVariant=Disabled  FdbkBlocksVariant=Forward  IdealPFdbkVariant=Disabled  SatFdbkVariant=Disabled  DerivativeFilterVariant=ContFilter  NVariant=InternalParameters  NCopyVariant=Disabled  FilterICVariant=InternalICsFilter  IntegratorICVariant=InternalICs  ExternalResetVariant=Disabled  TRSumVariant=Passthrough  SumFdbkVariant=Disabled  SumVariant=Sum_PID  TsampFilterVariant=InternalTs  TsampNgainVariant=Passthrough  TsampIntegralVariant=Disabled_SignalSpec  ExternalSaturationOutDataTypeStr=Inherit: Same as second input  DerivativeSourceVariant=ErrorSignal
  PID Controller (2DOF)5 : slpidlib/PID Controller (2DOF)  Controller=PID  Form=Parallel  TimeDomain=Continuous-time  UseExternalTs=off  SampleTime=-1  IntegratorMethod=Forward Euler  FilterMethod=Forward Euler  ControllerParametersSource=internal  P=6  I=1  UseKiTs=off  D=0  UseExternalDerivativeSource=off  N=100  UseFilter=on  b=1  c=1  TunerSelectOption=Transfer Function Based (PID Tuner App)  InitialConditionSource=internal  InitialConditionForIntegrator=0  InitialConditionForFilter=0  DifferentiatorICPrevScaledInput=0  ExternalReset=none  TrackingMode=off  Kt=1  LimitOutput=on  SatLimitsSource=internal  UpperSaturationLimit=30  LowerSaturationLimit=-30  LinearizeAsGain=on  AntiWindupMode=clamping  Kb=1  LimitIntegrator=off  UpperIntegratorSaturationLimit=inf  LowerIntegratorSaturationLimit=-inf  POutMin=[]  POutMax=[]  IOutMin=[]  IOutMax=[]  DOutMin=[]  DOutMax=[]  NOutMin=[]  NOutMax=[]  bOutMin=[]  bOutMax=[]  cOutMin=[]  cOutMax=[]  SumOutMin=[]  SumOutMax=[]  SaturationOutMin=[]  SaturationOutMax=[]  PParamMin=[]  PParamMax=[]  IParamMin=[]  IParamMax=[]  DParamMin=[]  DParamMax=[]  NParamMin=[]  NParamMax=[]  bParamMin=[]  bParamMax=[]  cParamMin=[]  cParamMax=[]  KbParamMin=[]  KbParamMax=[]  KtParamMin=[]  KtParamMax=[]  KbOutMin=[]  KbOutMax=[]  KtOutMin=[]  KtOutMax=[]  IntegratorOutMin=[]  IntegratorOutMax=[]  FilterOutMin=[]  FilterOutMax=[]  SumI1OutMin=[]  SumI1OutMax=[]  SumI2OutMin=[]  SumI2OutMax=[]  SumI3OutMin=[]  SumI3OutMax=[]  SumI4OutMin=[]  SumI4OutMax=[]  SumDOutMin=[]  SumDOutMax=[]  Sum1OutMin=[]  Sum1OutMax=[]  Sum2OutMin=[]  Sum2OutMax=[]  Sum3OutMin=[]  Sum3OutMax=[]  DifferentiatorOutMin=[]  DifferentiatorOutMax=[]  FilterDiffOutCoefMin=[]  FilterDiffOutCoefMax=[]  ReciprocalOutMin=[]  ReciprocalOutMax=[]  SumDenOutMin=[]  SumDenOutMax=[]  SumNumOutMin=[]  SumNumOutMax=[]  DivideOutMin=[]  DivideOutMax=[]  UdiffTsProdOutMin=[]  UdiffTsProdOutMax=[]  NTsProdOutMin=[]  NTsProdOutMax=[]  UintegralTsProdOutMin=[]  UintegralTsProdOutMax=[]  UngainTsProdOutMin=[]  UngainTsProdOutMax=[]  ClampingZeroOutDataTypeStr=Inherit: Inherit via back propagation  ClampingZeroOutMin=[]  ClampingZeroOutMax=[]  FilterDenConstantOutDataTypeStr=Inherit: Inherit via back propagation  FilterDenConstantOutMin=[]  FilterDenConstantOutMax=[]  PCopyOutDataTypeStr=Inherit: Inherit via back propagation  PCopyOutMin=[]  PCopyOutMax=[]  NCopyOutDataTypeStr=Inherit: Inherit via back propagation  NCopyOutMin=[]  NCopyOutMax=[]  IntegratorContinuousStateAttributes=''  IntegratorStateMustResolveToSignalObject=off  IntegratorRTWStateStorageClass=Auto  FilterContinuousStateAttributes=''  FilterStateMustResolveToSignalObject=off  FilterRTWStateStorageClass=Auto  ParallelPVariant=InternalParameters  IdealPVariant=Disabled  IVariant=InternalParameters  DVariant=InternalParameters  bVariant=InternalParameters  cVariant=InternalParameters  IntegratorVariant=Continuous  SatVariant=Enabled  AWVariant=ContClampingParallel  PCopyVariant=Disabled  TRVariant=Disabled  FdbkBlocksVariant=Forward  IdealPFdbkVariant=Disabled  SatFdbkVariant=Disabled  DerivativeFilterVariant=ContFilter  NVariant=InternalParameters  NCopyVariant=Disabled  FilterICVariant=InternalICsFilter  IntegratorICVariant=InternalICs  ExternalResetVariant=Disabled  TRSumVariant=Passthrough  SumFdbkVariant=Disabled  SumVariant=Sum_PID  TsampFilterVariant=InternalTs  TsampNgainVariant=Passthrough  TsampIntegralVariant=Disabled_SignalSpec  ExternalSaturationOutDataTypeStr=Inherit: Same as second input  DerivativeSourceVariant=ErrorSignal
  PID Controller (2DOF)6 : slpidlib/PID Controller (2DOF)  Controller=PID  Form=Parallel  TimeDomain=Continuous-time  UseExternalTs=off  SampleTime=-1  IntegratorMethod=Forward Euler  FilterMethod=Forward Euler  ControllerParametersSource=internal  P=6  I=1  UseKiTs=off  D=0  UseExternalDerivativeSource=off  N=100  UseFilter=on  b=1  c=1  TunerSelectOption=Transfer Function Based (PID Tuner App)  InitialConditionSource=internal  InitialConditionForIntegrator=0  InitialConditionForFilter=0  DifferentiatorICPrevScaledInput=0  ExternalReset=none  TrackingMode=off  Kt=1  LimitOutput=on  SatLimitsSource=internal  UpperSaturationLimit=30  LowerSaturationLimit=-30  LinearizeAsGain=on  AntiWindupMode=clamping  Kb=1  LimitIntegrator=off  UpperIntegratorSaturationLimit=inf  LowerIntegratorSaturationLimit=-inf  POutMin=[]  POutMax=[]  IOutMin=[]  IOutMax=[]  DOutMin=[]  DOutMax=[]  NOutMin=[]  NOutMax=[]  bOutMin=[]  bOutMax=[]  cOutMin=[]  cOutMax=[]  SumOutMin=[]  SumOutMax=[]  SaturationOutMin=[]  SaturationOutMax=[]  PParamMin=[]  PParamMax=[]  IParamMin=[]  IParamMax=[]  DParamMin=[]  DParamMax=[]  NParamMin=[]  NParamMax=[]  bParamMin=[]  bParamMax=[]  cParamMin=[]  cParamMax=[]  KbParamMin=[]  KbParamMax=[]  KtParamMin=[]  KtParamMax=[]  KbOutMin=[]  KbOutMax=[]  KtOutMin=[]  KtOutMax=[]  IntegratorOutMin=[]  IntegratorOutMax=[]  FilterOutMin=[]  FilterOutMax=[]  SumI1OutMin=[]  SumI1OutMax=[]  SumI2OutMin=[]  SumI2OutMax=[]  SumI3OutMin=[]  SumI3OutMax=[]  SumI4OutMin=[]  SumI4OutMax=[]  SumDOutMin=[]  SumDOutMax=[]  Sum1OutMin=[]  Sum1OutMax=[]  Sum2OutMin=[]  Sum2OutMax=[]  Sum3OutMin=[]  Sum3OutMax=[]  DifferentiatorOutMin=[]  DifferentiatorOutMax=[]  FilterDiffOutCoefMin=[]  FilterDiffOutCoefMax=[]  ReciprocalOutMin=[]  ReciprocalOutMax=[]  SumDenOutMin=[]  SumDenOutMax=[]  SumNumOutMin=[]  SumNumOutMax=[]  DivideOutMin=[]  DivideOutMax=[]  UdiffTsProdOutMin=[]  UdiffTsProdOutMax=[]  NTsProdOutMin=[]  NTsProdOutMax=[]  UintegralTsProdOutMin=[]  UintegralTsProdOutMax=[]  UngainTsProdOutMin=[]  UngainTsProdOutMax=[]  ClampingZeroOutDataTypeStr=Inherit: Inherit via back propagation  ClampingZeroOutMin=[]  ClampingZeroOutMax=[]  FilterDenConstantOutDataTypeStr=Inherit: Inherit via back propagation  FilterDenConstantOutMin=[]  FilterDenConstantOutMax=[]  PCopyOutDataTypeStr=Inherit: Inherit via back propagation  PCopyOutMin=[]  PCopyOutMax=[]  NCopyOutDataTypeStr=Inherit: Inherit via back propagation  NCopyOutMin=[]  NCopyOutMax=[]  IntegratorContinuousStateAttributes=''  IntegratorStateMustResolveToSignalObject=off  IntegratorRTWStateStorageClass=Auto  FilterContinuousStateAttributes=''  FilterStateMustResolveToSignalObject=off  FilterRTWStateStorageClass=Auto  ParallelPVariant=InternalParameters  IdealPVariant=Disabled  IVariant=InternalParameters  DVariant=InternalParameters  bVariant=InternalParameters  cVariant=InternalParameters  IntegratorVariant=Continuous  SatVariant=Enabled  AWVariant=ContClampingParallel  PCopyVariant=Disabled  TRVariant=Disabled  FdbkBlocksVariant=Forward  IdealPFdbkVariant=Disabled  SatFdbkVariant=Disabled  DerivativeFilterVariant=ContFilter  NVariant=InternalParameters  NCopyVariant=Disabled  FilterICVariant=InternalICsFilter  IntegratorICVariant=InternalICs  ExternalResetVariant=Disabled  TRSumVariant=Passthrough  SumFdbkVariant=Disabled  SumVariant=Sum_PID  TsampFilterVariant=InternalTs  TsampNgainVariant=Passthrough  TsampIntegralVariant=Disabled_SignalSpec  ExternalSaturationOutDataTypeStr=Inherit: Same as second input  DerivativeSourceVariant=ErrorSignal
  Pitch Angle Cmd [deg] : Constant  Value=0
  RPM0 : Constant  Value=5375
  Radians to Degrees : simulink_extras/Transformations/Radians to Degrees
  Sensors{1..7} (7 alike) : InportShadow
  Sum : Sum  Inputs=++|
  T/W_0 : Constant  Value=0.92
  Thrust-to-Weight Cmd [-] : Constant  Value=0
  Velocity Cmd [kts] : Constant  Value=0
  Vertical Velocity Cmd [m/s] : Constant  Value=0
  Yaw Rate Cmd [deg/s] : Constant  Value=0
  Yaw Rate Cmd [deg/s]1 : Constant  Value=0
  kts --> m/s : Gain  Gain=0.514444
  kts --> m/s1 : Gain  Gain=0.514444
  udir : Constant  Value=0
  ulat : Constant  Value=0
  ulon : Constant  Value=0
  RPM Cmds : Outport
  wires:
  PID Controller (2DOF)1/1 -> Mux2/1
  PID Controller (2DOF)/1 -> Mux2/2
  Mux2/1 -> MATLAB Function/1(UTrimVec)
  PID Controller (2DOF)3/1 -> MATLAB Function2/1(TW_Cmd)  "T/W Cmd"
  PID Controller (2DOF)2/1 -> Mux2/3
  MATLAB Function/1(U) -> RPM Cmds/1
  Sensors/1 -> Bus Selector/1
  Bus Selector/1 -> PID Controller (2DOF)/2  "<theta>"
  Gain3/1 -> Degrees to Radians/1
  Degrees to Radians/1 -> PID Controller (2DOF)/1
  Degrees to Radians1/1 -> PID Controller (2DOF)1/1
  Bus Selector1/1 -> PID Controller (2DOF)1/2  "<phi>"
  Sensors1/1 -> Bus Selector1/1
  PID Controller (2DOF)6/1 -> Degrees to Radians1/1
  Bus Selector2/1 -> PID Controller (2DOF)2/2  "<r>"
  Yaw Rate Cmd [deg/s]/1 -> Degrees to Radians2/1
  Degrees to Radians2/1 -> PID Controller (2DOF)2/1
  Sensors2/1 -> Bus Selector2/1
  PID Controller (2DOF)4/1 -> PID Controller (2DOF)3/1
  Sensors3/1 -> Bus Selector3/1
  Bus Selector3/1 -> PID Controller (2DOF)3/2  "<VV>"
  T/W_0/1 -> PID Controller (2DOF)3/3
  Constant/1 -> PID Controller (2DOF)3/4
  Altitude Cmd [ft]/1 -> Gain2/1
  Bus Selector4/1 -> Gain1/1  "<z>"
  Sensors4/1 -> Bus Selector4/1
  Gain1/1 -> PID Controller (2DOF)4/2
  Gain2/1 -> PID Controller (2DOF)4/1
  kts --> m/s/1 -> PID Controller (2DOF)5/1
  Velocity Cmd [kts]/1 -> kts --> m/s/1
  Sensors5/1 -> Bus Selector5/1
  Bus Selector5/1 -> PID Controller (2DOF)5/2  "<VFWD>"
  PID Controller (2DOF)5/1 -> Gain3/1
  Lateral Velocity Cmd [kts]/1 -> kts --> m/s1/1
  kts --> m/s1/1 -> PID Controller (2DOF)6/1
  Bus Selector6/1 -> PID Controller (2DOF)6/2  "<VLAT>"
  Sensors6/1 -> Bus Selector6/1
  MATLAB Function2/1(T_Cmd) -> MATLAB Function1/1(T_Cmd)
  Sum/1 -> MATLAB Function1/2(AOI)
  Constant2/1 -> MATLAB Function1/3(V_ms)
  Constant3/1 -> MATLAB Function1/5(delta_RPM)
  Constant5/1 -> MATLAB Function2/2(nProps)
  Constant6/1 -> Gain4/1
  Gain4/1 -> MATLAB Function2/3(Weight)
  [Atmos] -> Bus Selector7/1
  Bus Selector7/1 -> MATLAB Function1/4(rho)  "<rho (kg/m3)>"
  Constant1/1 -> Sum/2
  Sensors7/1 -> Bus Selector8/1
  Bus Selector8/1 -> Radians to Degrees/1  "<theta>"
  Radians to Degrees/1 -> Sum/1
  MATLAB Function1/1(RPM) -> Mux2/4

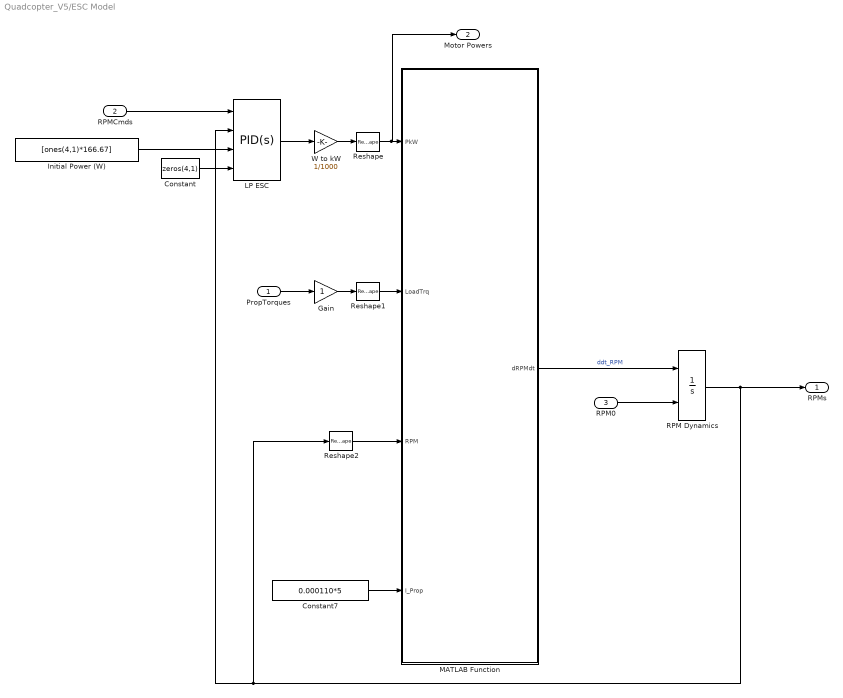
== system Quadcopter_V5/ESC Model ==
  PropTorques : Inport
  RPMCmds : Inport  Port=2
  RPM0 : Inport  Port=3
  Constant : Constant  Value=zeros(4,1)
  Constant7 : Constant  Value=0.000110*5
  Gain : Gain
  Initial Power (W) : Constant  Value=[ones(4,1)*166.67]
  LP ESC : slpidlib/PID Controller (2DOF)  Controller=PID  Form=Parallel  TimeDomain=Continuous-time  UseExternalTs=off  SampleTime=-1  IntegratorMethod=Forward Euler  FilterMethod=Forward Euler  ControllerParametersSource=internal  P=2  I=3  UseKiTs=off  D=0  UseExternalDerivativeSource=off  N=100  UseFilter=on  b=1  c=0  TunerSelectOption=Transfer Function Based (PID Tuner App)  InitialConditionSource=external  InitialConditionForIntegrator=0  InitialConditionForFilter=0  DifferentiatorICPrevScaledInput=0  ExternalReset=none  TrackingMode=off  Kt=1  LimitOutput=on  SatLimitsSource=internal  UpperSaturationLimit=500  LowerSaturationLimit=-500  LinearizeAsGain=on  AntiWindupMode=clamping  Kb=1  LimitIntegrator=off  UpperIntegratorSaturationLimit=inf  LowerIntegratorSaturationLimit=-inf  POutMin=[]  POutMax=[]  IOutMin=[]  IOutMax=[]  DOutMin=[]  DOutMax=[]  NOutMin=[]  NOutMax=[]  bOutMin=[]  bOutMax=[]  cOutMin=[]  cOutMax=[]  SumOutMin=[]  SumOutMax=[]  SaturationOutMin=[]  SaturationOutMax=[]  PParamMin=[]  PParamMax=[]  IParamMin=[]  IParamMax=[]  DParamMin=[]  DParamMax=[]  NParamMin=[]  NParamMax=[]  bParamMin=[]  bParamMax=[]  cParamMin=[]  cParamMax=[]  KbParamMin=[]  KbParamMax=[]  KtParamMin=[]  KtParamMax=[]  KbOutMin=[]  KbOutMax=[]  KtOutMin=[]  KtOutMax=[]  IntegratorOutMin=[]  IntegratorOutMax=[]  FilterOutMin=[]  FilterOutMax=[]  SumI1OutMin=[]  SumI1OutMax=[]  SumI2OutMin=[]  SumI2OutMax=[]  SumI3OutMin=[]  SumI3OutMax=[]  SumI4OutMin=[]  SumI4OutMax=[]  SumDOutMin=[]  SumDOutMax=[]  Sum1OutMin=[]  Sum1OutMax=[]  Sum2OutMin=[]  Sum2OutMax=[]  Sum3OutMin=[]  Sum3OutMax=[]  DifferentiatorOutMin=[]  DifferentiatorOutMax=[]  FilterDiffOutCoefMin=[]  FilterDiffOutCoefMax=[]  ReciprocalOutMin=[]  ReciprocalOutMax=[]  SumDenOutMin=[]  SumDenOutMax=[]  SumNumOutMin=[]  SumNumOutMax=[]  DivideOutMin=[]  DivideOutMax=[]  UdiffTsProdOutMin=[]  UdiffTsProdOutMax=[]  NTsProdOutMin=[]  NTsProdOutMax=[]  UintegralTsProdOutMin=[]  UintegralTsProdOutMax=[]  UngainTsProdOutMin=[]  UngainTsProdOutMax=[]  ClampingZeroOutDataTypeStr=Inherit: Inherit via back propagation  ClampingZeroOutMin=[]  ClampingZeroOutMax=[]  FilterDenConstantOutDataTypeStr=Inherit: Inherit via back propagation  FilterDenConstantOutMin=[]  FilterDenConstantOutMax=[]  PCopyOutDataTypeStr=Inherit: Inherit via back propagation  PCopyOutMin=[]  PCopyOutMax=[]  NCopyOutDataTypeStr=Inherit: Inherit via back propagation  NCopyOutMin=[]  NCopyOutMax=[]  IntegratorContinuousStateAttributes=''  IntegratorStateMustResolveToSignalObject=off  IntegratorRTWStateStorageClass=Auto  FilterContinuousStateAttributes=''  FilterStateMustResolveToSignalObject=off  FilterRTWStateStorageClass=Auto  ParallelPVariant=InternalParameters  IdealPVariant=Disabled  IVariant=InternalParameters  DVariant=InternalParameters  bVariant=InternalParameters  cVariant=InternalParameters  IntegratorVariant=Continuous  SatVariant=Enabled  AWVariant=ContClampingParallel  PCopyVariant=Disabled  TRVariant=Disabled  FdbkBlocksVariant=Forward  IdealPFdbkVariant=Disabled  SatFdbkVariant=Disabled  DerivativeFilterVariant=ContFilter  NVariant=InternalParameters  NCopyVariant=Disabled  FilterICVariant=ExternalICs  IntegratorICVariant=ExternalICs  ExternalResetVariant=Disabled  TRSumVariant=Passthrough  SumFdbkVariant=Disabled  SumVariant=Sum_PID  TsampFilterVariant=InternalTs  TsampNgainVariant=Passthrough  TsampIntegralVariant=Disabled_SignalSpec  ExternalSaturationOutDataTypeStr=Inherit: Same as second input  DerivativeSourceVariant=ErrorSignal
  MATLAB Function : MATLAB Function  TreatAsAtomicUnit=on
  RPM Dynamics : Integrator  InitialConditionSource=external  LimitOutput=on  UpperSaturationLimit=12000  LowerSaturationLimit=0
  Reshape : Reshape  OutputDimensionality=Row vector (2-D)
  Reshape1 : Reshape  OutputDimensionality=Row vector (2-D)
  Reshape2 : Reshape  OutputDimensionality=Column vector (2-D)
  W to kW : Gain  Gain=1/1000
  RPMs : Outport
  Motor Powers : Outport  Port=2
  wires:
  RPM0/1 -> RPM Dynamics/2
  MATLAB Function/1(dRPMdt) -> RPM Dynamics/1  "ddt_RPM"
  RPM Dynamics/1 -> RPMs/1, LP ESC/2, Reshape2/1
  Constant/1 -> LP ESC/4
  Constant7/1 -> MATLAB Function/4(I_Prop)
  Reshape/1 -> Motor Powers/1, MATLAB Function/1(PkW)
  Reshape1/1 -> MATLAB Function/2(LoadTrq)
  LP ESC/1 -> W to kW/1
  Reshape2/1 -> MATLAB Function/3(RPM)
  PropTorques/1 -> Gain/1
  W to kW/1 -> Reshape/1
  Initial Power (W)/1 -> LP ESC/3
  RPMCmds/1 -> LP ESC/1
  Gain/1 -> Reshape1/1

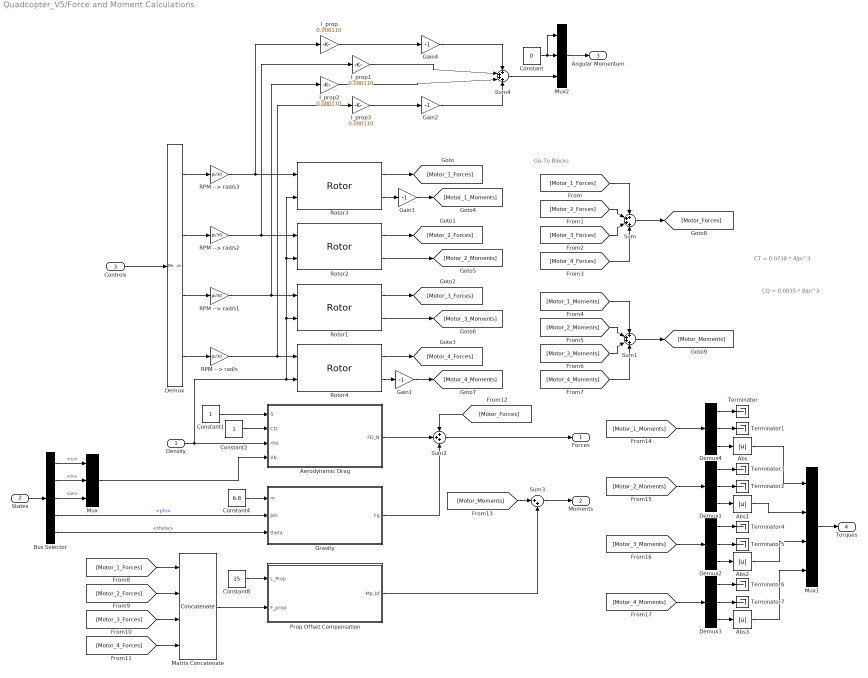
== system Quadcopter_V5/Force and Moment Calculations ==
  note: Go-To Blocks
  note: CQ = 0.0035 * 8/pi^3
  note: CT = 0.0738 * 4/pi^3
  Density : Inport
  States : Inport  Port=2
  Controls : Inport  Port=3
  Abs{,1..3} (4 alike) : Abs  SaturateOnIntegerOverflow=off
  Aerodynamic Drag : MATLAB Function  TreatAsAtomicUnit=on
  Bus Selector : BusSelector  OutputSignals=u,v,w,phi,theta
  Constant : Constant  Value=0
  Constant1 : Constant
  Constant2 : Constant
  Constant4 : Constant  Value=6.8
  Constant8 : Constant  Value=15
  Demux : Demux
  Demux{1..4} (4 alike) : Demux  Outputs=3
  Gain{1..4} (4 alike) : Gain  Gain=-1
  Gravity : MATLAB Function  TreatAsAtomicUnit=on
  I_prop{,1..3} (4 alike) : Gain  Gain=0.000110
  Matrix Concatenate : Concatenate  NumInputs=4  Mode=Multidimensional array  ConcatenateDimension=2
  Mux : Mux  Inputs=3
  Mux1 : Mux
  Mux2 : Mux  Inputs=3
  Prop Offset Compensation : MATLAB Function  TreatAsAtomicUnit=on
  RPM --> rad/s{,1..3} (4 alike) : Gain  Gain=pi/30
  Rotor{1..4} (4 alike) : aerolibpropulsion2/Rotor  units=Metric (MKS)  modelMode=Without flap effects  blockSelect=Single  config=Quadcopter X  Nr=1  l=0.0624  h=-0.0159  Arm=[0;0;0]  Nb=2  CTcheck=off  CT=0.0862 * 4/pi^3  CQ=0.0043 * 8/pi^3  CTout=off  R=15/39.37/2  c=0.0080  e=0  clalpha=5.5  gamma=0.6051  twistType=Linear  theta0=0.2548  theta1=-0.1361  thetaTip=0.1018  Vb=[0;0;0]  pqr=[0;0;0]
      settings: LibrarySourceBlock=aerolibrotor/Rotor
  Sum : Sum  Inputs=++++
  Sum1 : Sum  Inputs=++++
  Sum2 : Sum  Inputs=+++
  Sum3 : Sum  Inputs=|++
  Sum4 : Sum  Inputs=++++
  Terminator{,1..7} (8 alike) : Terminator
  Forces : Outport
  Moments : Outport  Port=2
  Angular Momentum : Outport  Port=3
  Torques : Outport  Port=4
  wires:
  RPM --> rad/s3/1 -> I_prop/1, Rotor3/1
  Constant4/1 -> Gravity/1(m)
  Constant1/1 -> Aerodynamic Drag/1(S)
  Rotor3/1 -> [Motor_1_Forces]
  RPM --> rad/s/1 -> Rotor4/1, I_prop3/1
  [Motor_Forces] -> Sum2/1
  Sum/1 -> [Motor_Forces]
  RPM --> rad/s2/1 -> Rotor2/1, I_prop1/1
  Rotor4/1 -> [Motor_4_Forces]
  [Motor_2_Forces] -> Sum/2
  Gain3/1 -> [Motor_1_Moments]
  [Motor_3_Forces] -> Sum/3
  Rotor1/2 -> [Motor_3_Moments]
  Rotor1/1 -> [Motor_3_Forces]
  [Motor_4_Forces] -> Sum/4
  Rotor2/1 -> [Motor_2_Forces]
  Rotor2/2 -> [Motor_2_Moments]
  Constant8/1 -> Prop Offset Compensation/1(L_Prop)
  Density/1 -> Aerodynamic Drag/3(rho), Rotor4/2, Rotor1/2, Rotor2/2, Rotor3/2
  Matrix Concatenate/1 -> Prop Offset Compensation/2(F_prop)
  Rotor3/2 -> Gain3/1
  [Motor_4_Moments] -> Sum1/4
  Mux/1 -> Aerodynamic Drag/4(Vb)
  Sum3/1 -> Moments/1
  RPM --> rad/s1/1 -> Rotor1/1, I_prop2/1
  [Motor_1_Forces] -> Matrix Concatenate/1
  [Motor_3_Forces] -> Matrix Concatenate/3
  [Motor_1_Moments] -> Sum1/1
  Gain1/1 -> [Motor_4_Moments]
  [Motor_3_Moments] -> Sum1/3
  Aerodynamic Drag/1(FD_N) -> Sum2/2
  [Motor_2_Moments] -> Sum1/2
  [Motor_4_Forces] -> Matrix Concatenate/4
  [Motor_1_Forces] -> Sum/1
  [Motor_2_Forces] -> Matrix Concatenate/2
  Sum1/1 -> [Motor_Moments]
  Constant2/1 -> Aerodynamic Drag/2(CD)
  Prop Offset Compensation/1(Mp_bf) -> Sum3/2
  Rotor4/2 -> Gain1/1
  Gravity/1(Fg) -> Sum2/3
  [Motor_Moments] -> Sum3/1
  Sum2/1 -> Forces/1
  States/1 -> Bus Selector/1
  Bus Selector/5 -> Gravity/3(theta)  "<theta>"
  Bus Selector/4 -> Gravity/2(phi)  "<phi>"
  Bus Selector/1 -> Mux/1  "<u>"
  Bus Selector/2 -> Mux/2  "<v>"
  Bus Selector/3 -> Mux/3  "<w>"
  Demux/4 -> RPM --> rad/s/1
  Demux/3 -> RPM --> rad/s1/1
  Demux/2 -> RPM --> rad/s2/1
  Demux/1 -> RPM --> rad/s3/1
  Controls/1 -> Demux/1
  [Motor_1_Moments] -> Demux4/1
  [Motor_2_Moments] -> Demux1/1
  [Motor_3_Moments] -> Demux2/1
  [Motor_4_Moments] -> Demux3/1
  Demux4/1 -> Terminator/1
  Demux4/2 -> Terminator1/1
  Demux1/2 -> Terminator2/1
  Demux1/1 -> Terminator3/1
  Demux2/1 -> Terminator4/1
  Demux2/2 -> Terminator5/1
  Demux3/1 -> Terminator6/1
  Demux3/2 -> Terminator7/1
  Demux4/3 -> Abs/1
  Demux1/3 -> Abs1/1
  Demux3/3 -> Abs3/1
  Demux2/3 -> Abs2/1
  Abs/1 -> Mux1/1
  Abs1/1 -> Mux1/2
  Abs2/1 -> Mux1/3
  Abs3/1 -> Mux1/4
  Mux1/1 -> Torques/1
  Sum4/1 -> Mux2/3
  I_prop/1 -> Gain4/1
  I_prop1/1 -> Sum4/2
  I_prop2/1 -> Sum4/3
  I_prop3/1 -> Gain2/1
  Gain2/1 -> Sum4/4
  Gain4/1 -> Sum4/1
  Mux2/1 -> Angular Momentum/1
  Constant/1 -> Mux2/1, Mux2/2
